simulink model "exsim"  (R2025a)
settings: Solver=VariableStepDiscrete  StartTime=0.0  StopTime=1.2  RelTol=1e-3  EnableMultiTasking=on
InitFcn:
  | % Change group to the index of your group
  | group = 2;
  | [u,c] = T2data(group);
values from neighbouring files (symbols this model uses):
  D = find_D(D_coarse - 10, 1, D_coarse + 10)    [T2.m]    (also in T3.m = 39)
  L = find_L(max(1, L_coarse - 10), 1, L_coarse + 10)    [T2.m]    (also in T3.m = 37)
libraries: simulink x5, dspsrcs4 x2, dspadpt3 x1
settings Model: Creator=psangi  LastModifiedBy=JONIK
settings SolverCC: AlgebraicLoopSolver=TrustRegion
settings DataIOCC: LimitDataPoints=on  SaveFormat=Array  SignalLoggingSaveFormat=ModelDataLogs  ReturnWorkspaceOutputs=off
settings OptimizationCC: ExpressionDepthLimit=2147483647.0  InitFltsAndDblsToZero=on  LifeSpan=inf
settings DebuggingCC: UnderspecifiedInitializationDetection=Classic  MergeDetectMultiDrivingBlocksExec=none  SolverPrmCheckMsg=warning  FcnCallInpInsideContextMsg=warning  UnconnectedInputMsg=warning  UnconnectedOutputMsg=warning  UnconnectedLineMsg=warning  StateNameClashWarn=warning  SFUnexpectedBacktrackingDiag=warning  SFNoUnconditionalDefaultTransitionDiag=warning  SFExecutionAtInitializationDiag=none  ArithmeticOperatorsInVariantConditions=warning
settings HardwareCC: ProdBitPerPointer=32.0  ProdBitPerSizeT=32.0  ProdBitPerPtrDiffT=32.0  ProdLargestAtomicFloat=None  ProdIntDivRoundTo=Undefined  ProdEndianess=Unspecified  ProdWordSize=32.0  ProdHWDeviceType=32-bit Generic
settings ModelReferenceCC: EnableRefExpFcnMdlSchedulingChecks=on  PropagateSignalLabelsOutOfModel=off
settings SFSimCC: SimUseLocalCustomCode=off  CustomCodeUndefinedFunction=UseInterfaceOnly
settings RTWCC: RTWUseLocalCustomCode=off  GPUComputeCapability=3.5
settings CodeAppCC: StateflowObjectComments=on
settings GRTTargetCC: TargetLangStandard=C89/C90 (ANSI)  CombineOutputUpdateFcns=off  GRTInterface=on
settings ConfigComp: CovMetricSettings=dw  CovSaveCumulativeToWorkspaceVar=on  CovSaveSingleToWorkspaceVar=on  CovExternalEMLEnable=off

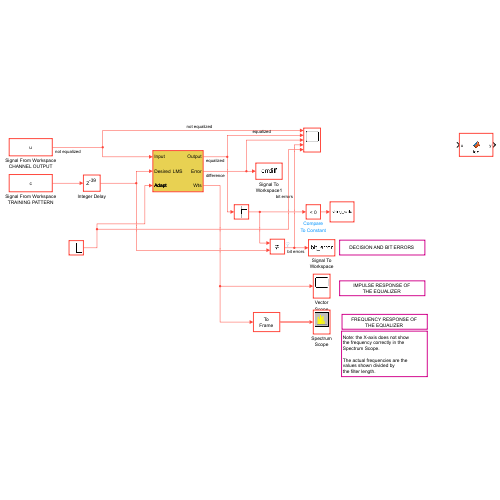
[thumbnail: Simulink's stored preview of the top-level diagram]
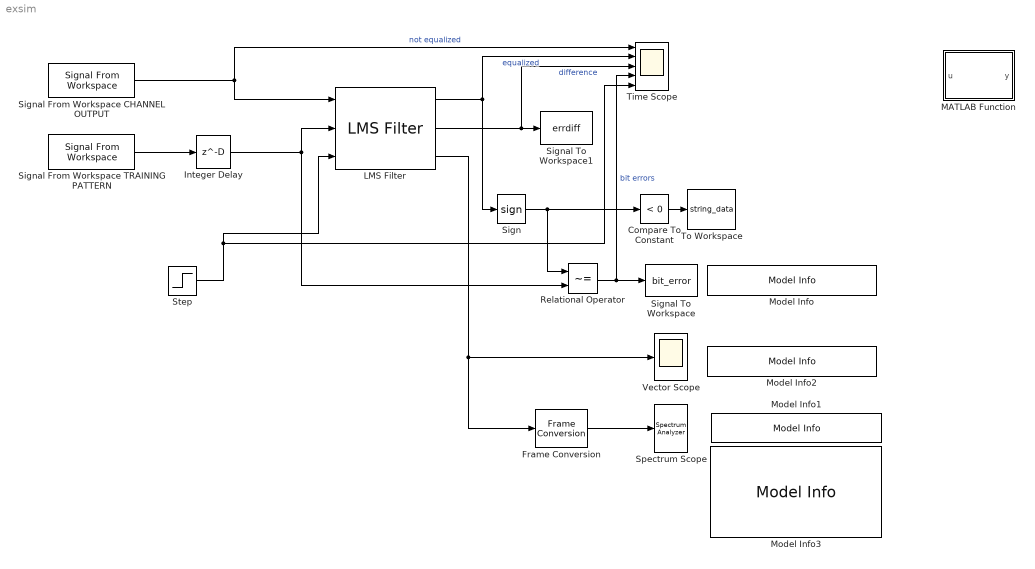
== system exsim ==
  Compare To Constant : simulink/Logic and Bit Operations/Compare To Constant  relop=<  const=0  OutDataTypeStr=boolean
  Frame Conversion : FrameConversion
  Integer Delay : Delay  DelayLength=D  InitialCondition=0
  LMS Filter : dspadpt3/LMS Filter  Algo=LMS  L=L  stepflag=Dialog  mu=step_size  leakage=1.0  ic=0  Adapt=on  resetflag=None  weights=on  addnparflag=off  roundingMode=Floor  overflowMode=off  secondCoeffMode=Binary point scaling  secondCoeffWordLength=2  secondCoeffFracLength=15  prodOutput2Mode=Binary point scaling  prodOutput2FracLength=20  prodOutput3Mode=Binary point scaling  prodOutput3FracLength=20  prodOutput4Mode=Binary point scaling  prodOutput4FracLength=20  quotientMode=Binary point scaling  quotientFracLength=20  accum2Mode=Binary point scaling  accum2FracLength=20
  MATLAB Function : MATLAB Function  TreatAsAtomicUnit=on
  Model Info : simulink/Model-Wide Utilities/Model Info  Frame=on  DisplayStringWithTags=DECISION AND BIT ERRORS  HorizontalTextAlignment=Center  LeftAlignmentValue=0.5
  Model Info1 : simulink/Model-Wide Utilities/Model Info  Frame=on  DisplayStringWithTags=FREQUENCY RESPONSE OF THE EQUALIZER  HorizontalTextAlignment=Center  LeftAlignmentValue=0.5
  Model Info2 : simulink/Model-Wide Utilities/Model Info  Frame=on  DisplayStringWithTags=IMPULSE RESPONSE OF THE EQUALIZER  HorizontalTextAlignment=Center  LeftAlignmentValue=0.5
  Model Info3 : simulink/Model-Wide Utilities/Model Info  Frame=on  DisplayStringWithTags=|  HorizontalTextAlignment=Left  LeftAlignmentValue=0.02
      | Note: the X-axis does not show
      | the frequency correctly in the
      | Spectrum Scope.
      | 
      | The actual frequencies are the
      | values shown divided by
      | the filter length.
  Relational Operator : RelationalOperator  Operator=~=  OutDataTypeStr=boolean  InputSameDT=off
  Sign : Signum
  Signal From Workspace CHANNEL OUTPUT : dspsrcs4/Signal From Workspace  X=u  Ts=1/10000  nsamps=1  OutputAfterFinalValue=Setting to zero  ignoreOrWarnInputAndFrameLengths=off  OutputFrames=on
  Signal From Workspace TRAINING PATTERN : dspsrcs4/Signal From Workspace  X=c  Ts=1/10000  nsamps=1  OutputAfterFinalValue=Setting to zero  ignoreOrWarnInputAndFrameLengths=off  OutputFrames=on
  Signal To Workspace : ToWorkspace  VariableName=bit_error  SampleTime=-1
  Signal To Workspace1 : ToWorkspace  VariableName=errdiff  SampleTime=-1
  Spectrum Scope : SpectrumAnalyzer  WindowPosition=[1992.000000,134.000000,1206.000000,300.000000,]  Visible=on  ScopeFrameLocation=window  Method=Welch  SampleRate=4000000  FFTLength=128  Span=350000  StartFrequency=-175000  StopFrequency=175000  OverlapPercent=80  AveragingMethod=Running  SpectralAverages=10  YLimits=[-144.9250984130807 18.465708213818573]  AllowFFTLengthLessThanSamplesPerUpdate=on  DefaultConfigurationName=spbscopes.SpectrumAnalyzerBlockCfg  IsFrequencyInputMode=0  FrequencyVectorPort=0  FrequencyVectorFromPort=0  FrequencyInputRBWPort=0  FrequencyInputRBWFromPort=0
      settings: OpenAtSimulationStart=off
  Step : Step  Before=1  After=0  SampleTime=1/10000
  Time Scope : Scope  NumInputPorts=5
      settings: ActiveDisplayYMinimum=-1.1727727713718925  ActiveDisplayYMaximum=1.3996072918903206  DataLoggingSaveFormat=Structure
  To Workspace : ToWorkspace  VariableName=string_data  SampleTime=-1
  Vector Scope : Scope
      settings: TimeSpan=One frame period  ActiveDisplayYMinimum=-3.7310894813048492  ActiveDisplayYMaximum=7.2116653690248693  YLabel=Amplitude  DataLoggingSaveFormat=Array
  wires:
  Signal From Workspace TRAINING PATTERN/1 -> Integer Delay/1
  Signal From Workspace CHANNEL OUTPUT/1 -> LMS Filter/1, Time Scope/1  "not equalized"
  Integer Delay/1 -> LMS Filter/2, Relational Operator/2
  LMS Filter/1 -> Sign/1, Time Scope/2  "equalized"
  Sign/1 -> Compare To Constant/1, Relational Operator/1
  Relational Operator/1 -> Signal To Workspace/1, Time Scope/4  "bit errors"
  LMS Filter/2 -> Signal To Workspace1/1, Time Scope/3  "difference"
  LMS Filter/3 -> Vector Scope/1, Frame Conversion/1
  Frame Conversion/1 -> Spectrum Scope/1
  Step/1 -> Time Scope/5, LMS Filter/3
  Compare To Constant/1 -> To Workspace/1

== matlab function exsim/MATLAB Function ==
  data: u input; y output
function y = fcn(u)

persistent idx
persistent byte

if isempty(idx)
    idx = 1;
    byte = zeros(1, 7, 'uint8');
end

byte(idx) = u;
idx = idx + 1;

y = zeros(1, 7, 'uint8');

if idx == 7
    y = uint8(byte);
    idx = 1;
    byte(:) = 0;
end
